simulink model "Verifica_HINF_11032026"  (R2025b)
settings: Solver=VariableStepAuto  StartTime=0.0  StopTime=25.0  RelTol=1e-3
libraries: cstblocks x3
settings Model: Creator=salvo  LastModifiedBy=salvo

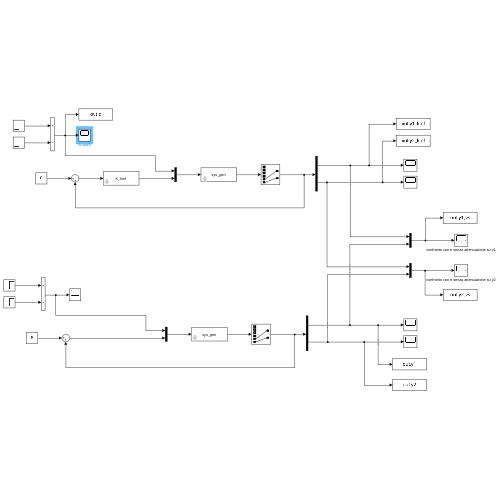
[thumbnail: Simulink's stored preview of the top-level diagram]
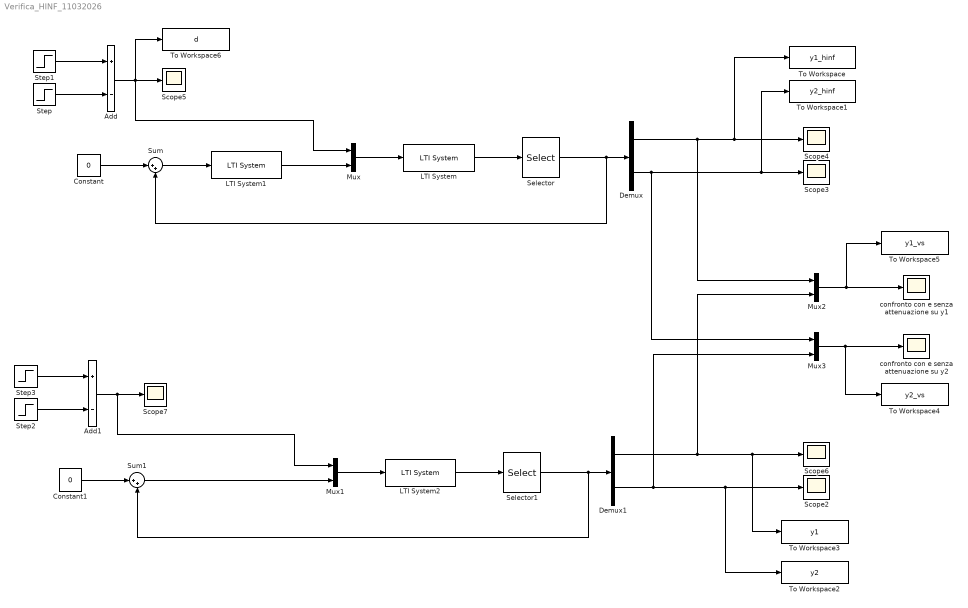
== system Verifica_HINF_11032026 ==
  Add : Sum  Inputs=+-
  Add1 : Sum  Inputs=+-
  Constant : Constant  Value=0
  Constant1 : Constant  Value=0
  Demux : Demux  Outputs=2
  Demux1 : Demux  Outputs=2
  LTI System : cstblocks/LTI System  sys=sys_gen  IC=[]  PadeOrder=0
  LTI System1 : cstblocks/LTI System  sys=K_hinf  IC=[]  PadeOrder=0
  LTI System2 : cstblocks/LTI System  sys=sys_gen  IC=[]  PadeOrder=0
  Mux{,1..3} (4 alike) : Mux  Inputs=2
  Scope{2..7} (6 alike) : Scope
      Scope2 settings: ActiveDisplayYMinimum=-2.2930353132593959  ActiveDisplayYMaximum=2.7558317357774578
      Scope3 settings: ActiveDisplayYMinimum=-2.2930353132593959  ActiveDisplayYMaximum=2.7558317357774578  DataLoggingVariableName=ScopeData2
      Scope4 settings: ActiveDisplayYMinimum=-0.60313892615814235  ActiveDisplayYMaximum=2.1769794267283817  DataLoggingVariableName=ScopeData3
      Scope5 settings: ActiveDisplayYMinimum=-6.2499999999999982  ActiveDisplayYMaximum=56.25  DataLoggingVariableName=ScopeData4
      Scope6 settings: ActiveDisplayYMinimum=-1.5651824919841739  ActiveDisplayYMaximum=0.1396281134462779  DataLoggingVariableName=ScopeData5
      Scope7 settings: ActiveDisplayYMinimum=-16.776057459193559  ActiveDisplayYMaximum=18.401453107193444  DataLoggingVariableName=ScopeData6
  Selector : Selector  InputPortWidth=6  IndexOptions=Index vector (dialog)  Indices=[5 6]  OutputSizes=1
  Selector1 : Selector  InputPortWidth=6  IndexOptions=Index vector (dialog)  Indices=[5 6]  OutputSizes=1
  Step : Step  Time=12  After=50  SampleTime=0
  Step1 : Step  Time=10  After=50  SampleTime=0
  Step2 : Step  Time=12  After=50  SampleTime=0
  Step3 : Step  Time=10  After=50  SampleTime=0
  Sum : Sum  Inputs=|++
  Sum1 : Sum  Inputs=|++
  To Workspace : ToWorkspace  VariableName=y1_hinf  SaveFormat=Timeseries  SampleTime=-1
  To Workspace1 : ToWorkspace  VariableName=y2_hinf  SaveFormat=Timeseries  SampleTime=-1
  To Workspace2 : ToWorkspace  VariableName=y2  SaveFormat=Timeseries  SampleTime=-1
  To Workspace3 : ToWorkspace  VariableName=y1  SaveFormat=Timeseries  SampleTime=-1
  To Workspace4 : ToWorkspace  VariableName=y2_vs  SaveFormat=Timeseries  SampleTime=-1
  To Workspace5 : ToWorkspace  VariableName=y1_vs  SaveFormat=Timeseries  SampleTime=-1
  To Workspace6 : ToWorkspace  VariableName=d  SaveFormat=Timeseries  SampleTime=-1
  confronto con e senza attenuazione su y1 : Scope
      settings: ActiveDisplayYMinimum=-1.6762724162259555  ActiveDisplayYMaximum=3.3658969074793275
  confronto con e senza attenuazione su y2 : Scope
      settings: ActiveDisplayYMinimum=-2.2930353132593959  ActiveDisplayYMaximum=2.7558317357774578  DataLoggingVariableName=ScopeData7
  wires:
  Mux/1 -> LTI System/1
  LTI System1/1 -> Mux/2
  Constant/1 -> Sum/1
  Sum/1 -> LTI System1/1
  LTI System/1 -> Selector/1
  Selector/1 -> Demux/1, Sum/2
  Demux/2 -> To Workspace1/1, Scope3/1, Mux3/1
  Demux/1 -> Scope4/1, To Workspace/1, Mux2/1
  Step/1 -> Add/2
  Step1/1 -> Add/1
  Add/1 -> To Workspace6/1, Scope5/1, Mux/1
  LTI System2/1 -> Selector1/1
  Selector1/1 -> Demux1/1, Sum1/2
  Demux1/1 -> To Workspace3/1, Scope6/1, Mux2/2
  Demux1/2 -> To Workspace2/1, Scope2/1, Mux3/2
  Sum1/1 -> Mux1/2
  Constant1/1 -> Sum1/1
  Step3/1 -> Add1/1
  Step2/1 -> Add1/2
  Mux1/1 -> LTI System2/1
  Add1/1 -> Scope7/1, Mux1/1
  Mux2/1 -> confronto con e senza attenuazione su y1/1, To Workspace5/1
  Mux3/1 -> To Workspace4/1, confronto con e senza attenuazione su y2/1
